simulink model "My_Model"  (R2022a)
settings: Solver=VariableStepAuto  StartTime=0.0  StopTime=10.0  RelTol=1e-3
libraries: neural x1294, spsSeriesRLCBranchLib x16, spsDiodeLib x14, spsMosfetLib x9, spsVoltageMeasurementLib x9, powerlib_extras x8, spsThreePhaseVIMeasurementLib x7, spsCurrentMeasurementLib x4, spsPVArrayLib x4, spsPWMGeneratorDCDCLib x4, spsTHDLib x4, spsThreePhaseParallelRLCBranchLib x3
(part 37 of 41)

== system My_Model/VSC Control/Current Regulator/7 layer network/Layer 4/LW{4,2} ==
  "ad{4,2}" : Inport  PortDimensions=10
      mask Display: e = 0.06;c1 = [120 230 180]/255;c2 = ([120 230 180]+0)/(256+128);c3 = ([120 230 180]+128)/(256+128);patch([0 1 1 0],[0 0 1 1],c1);patch([0 1 1 1-e 1-e 0+e],[0 0 1 1-e 0+e 0+e],c2);patch([0 0 1 1-e 0+e 0+e],[0 1 1 1-e 1-e 0+e],c3);plot([0 1 1 0 0],[0 0 1 1 0]);
  "IW{4,2}(1,:)'" : Constant  Value=[-0.060828921629580597063569058491339092142879962921142578125;0.775373578077013458909050314105115830898284912109375;-1.4812195216760304372627388147520832717418670654296875;1.4414249293693222053747149402624927461147308349609375;-0.600183260490783521134972033905796706676483154296875;-1.0932491360089870990890403845696710050106048583984375;-1.5989219798784224391141606247401796281337738037109375;0.83967493194491271690793610105174593627452850341796875;-1.416112923115345978430923423729836940765380859375;0.90341843686185929751530920839286409318447113037109375]
      mask Display: e = 0.06;c1 = [120 150 230]/255;c2 = ([120 150 230]+0)/383;c3 = ([120 150 230]+128)/383;patch([0 1 1 0],[0 0 1 1],c1);patch([0 1 1 1-e 1-e 0+e],[0 0 1 1-e 0+e 0+e],c2);patch([0 0 1 1-e 0+e 0+e],[0 1 1 1-e 1-e 0+e],c3);plot([0 1 1 0 0],[0 0 1 1 0]);disp('weights');
  "IW{4,2}(10,:)'" : Constant  Value=[0.310879887578999980490834786905907094478607177734375;1.7639693187841471999632858569384552538394927978515625;-0.818751635144346234795875716372393071651458740234375;0.81506969070432278012816595946787856519222259521484375;-1.6295109527652282821463813888840377330780029296875;-0.12293699794713031092641131181153468787670135498046875;-0.72363404737931935617467615884379483759403228759765625;-0.790138494286973358526893207454122602939605712890625;-1.4200799342452998796915153434383682906627655029296875;0.52091465079437615504076575234648771584033966064453125]
      mask Display: e = 0.06;c1 = [120 150 230]/255;c2 = ([120 150 230]+0)/383;c3 = ([120 150 230]+128)/383;patch([0 1 1 0],[0 0 1 1],c1);patch([0 1 1 1-e 1-e 0+e],[0 0 1 1-e 0+e 0+e],c2);patch([0 0 1 1-e 0+e 0+e],[0 1 1 1-e 1-e 0+e],c3);plot([0 1 1 0 0],[0 0 1 1 0]);disp('weights');
  "IW{4,2}(11,:)'" : Constant  Value=[1.217143736034584922123258365900255739688873291015625;0.981955089023607730069898025249131023883819580078125;0.1461353992399598566986895775698940269649028778076171875;0.9371123464038502159922927603474818170070648193359375;-1.095913271537847233361162579967640340328216552734375;1.5274566495244739083858576123020611703395843505859375;-1.586484384110760981201337926904670894145965576171875;0.7160108429212599379098946883459575474262237548828125;0.450020087913313882044263891657465137541294097900390625;0.011825737849426455616796971526127890683710575103759765625]
      mask Display: e = 0.06;c1 = [120 150 230]/255;c2 = ([120 150 230]+0)/383;c3 = ([120 150 230]+128)/383;patch([0 1 1 0],[0 0 1 1],c1);patch([0 1 1 1-e 1-e 0+e],[0 0 1 1-e 0+e 0+e],c2);patch([0 0 1 1-e 0+e 0+e],[0 1 1 1-e 1-e 0+e],c3);plot([0 1 1 0 0],[0 0 1 1 0]);disp('weights');
  "IW{4,2}(12,:)'" : Constant  Value=[1.324541573219643719738769505056552588939666748046875;0.277920776504625433034334491821937263011932373046875;0.718328783591281716525145384366624057292938232421875;-1.42965367074923843659917110926471650600433349609375;0.58329551863306094983130378750502131879329681396484375;-1.3283837730520866582395456134690903127193450927734375;-0.71009288846986395871141439783968962728977203369140625;0.22086308386329200903475111772422678768634796142578125;-0.56919723421407286689799320811289362609386444091796875;-1.1498144669477603496687834194744937121868133544921875]
      mask Display: e = 0.06;c1 = [120 150 230]/255;c2 = ([120 150 230]+0)/383;c3 = ([120 150 230]+128)/383;patch([0 1 1 0],[0 0 1 1],c1);patch([0 1 1 1-e 1-e 0+e],[0 0 1 1-e 0+e 0+e],c2);patch([0 0 1 1-e 0+e 0+e],[0 1 1 1-e 1-e 0+e],c3);plot([0 1 1 0 0],[0 0 1 1 0]);disp('weights');
  "IW{4,2}(13,:)'" : Constant  Value=[1.628084866678424447172801592387259006500244140625;1.46608398126954941886879169032908976078033447265625;-0.03245388683525977924215766279303352348506450653076171875;1.181646003765824293196828875807113945484161376953125;-0.641876045468599887300342743401415646076202392578125;0.82068797136729421115575178191647864878177642822265625;-1.56047384777860198568077976233325898647308349609375;-0.351567530724675225695108338186400942504405975341796875;0.54855116014444627037249802015139721333980560302734375;0.91871473917374724127427043640636838972568511962890625]
      mask Display: e = 0.06;c1 = [120 150 230]/255;c2 = ([120 150 230]+0)/383;c3 = ([120 150 230]+128)/383;patch([0 1 1 0],[0 0 1 1],c1);patch([0 1 1 1-e 1-e 0+e],[0 0 1 1-e 0+e 0+e],c2);patch([0 0 1 1-e 0+e 0+e],[0 1 1 1-e 1-e 0+e],c3);plot([0 1 1 0 0],[0 0 1 1 0]);disp('weights');
  "IW{4,2}(14,:)'" : Constant  Value=[-1.7329463683664869666500862877001054584980010986328125;0.2741436029171386845604274640209041535854339599609375;0.11238014359429461530570648619686835445463657379150390625;1.4837327723600723938801593249081633985042572021484375;1.356169480732644760934135774732567369937896728515625;0.8085467563784864974962829364812932908535003662109375;0.019157902600305108664624498260309337638318538665771484375;-1.519400622506951403778430176316760480403900146484375;0.839192151249030349191571076516993343830108642578125;-1.3888742432581280272785306806326843798160552978515625]
      mask Display: e = 0.06;c1 = [120 150 230]/255;c2 = ([120 150 230]+0)/383;c3 = ([120 150 230]+128)/383;patch([0 1 1 0],[0 0 1 1],c1);patch([0 1 1 1-e 1-e 0+e],[0 0 1 1-e 0+e 0+e],c2);patch([0 0 1 1-e 0+e 0+e],[0 1 1 1-e 1-e 0+e],c3);plot([0 1 1 0 0],[0 0 1 1 0]);disp('weights');
  "IW{4,2}(15,:)'" : Constant  Value=[1.2557485514732544817917414547991938889026641845703125;-1.7036258946208195919069794399547390639781951904296875;-0.1776350386540186676587183001174707897007465362548828125;1.68161376417911156977424980141222476959228515625;-1.33123786422297296638816987979225814342498779296875;0.22183289060876243414810460308217443525791168212890625;0.92045836890086685233569596675806678831577301025390625;0.9665236347790635562660099822096526622772216796875;0.31881726521650388672668441358837299048900604248046875;-0.7597052386250791045085861696861684322357177734375]
      mask Display: e = 0.06;c1 = [120 150 230]/255;c2 = ([120 150 230]+0)/383;c3 = ([120 150 230]+128)/383;patch([0 1 1 0],[0 0 1 1],c1);patch([0 1 1 1-e 1-e 0+e],[0 0 1 1-e 0+e 0+e],c2);patch([0 0 1 1-e 0+e 0+e],[0 1 1 1-e 1-e 0+e],c3);plot([0 1 1 0 0],[0 0 1 1 0]);disp('weights');
  "IW{4,2}(16,:)'" : Constant  Value=[0.383590307363950333563451522422838024795055389404296875;-1.441254533680973448639406342408619821071624755859375;-1.404217028320909665950466660433448851108551025390625;1.378999030353992960584719185135327279567718505859375;1.8023155948177276286514825187623500823974609375;-1.17934167700769165776364388875663280487060546875;0.46513754528094886087075110481237061321735382080078125;-0.61955378906156199914079252266674302518367767333984375;0.87675658573421488828358860700973309576511383056640625;-1.0257452924889649548134684664546512067317962646484375]
      mask Display: e = 0.06;c1 = [120 150 230]/255;c2 = ([120 150 230]+0)/383;c3 = ([120 150 230]+128)/383;patch([0 1 1 0],[0 0 1 1],c1);patch([0 1 1 1-e 1-e 0+e],[0 0 1 1-e 0+e 0+e],c2);patch([0 0 1 1-e 0+e 0+e],[0 1 1 1-e 1-e 0+e],c3);plot([0 1 1 0 0],[0 0 1 1 0]);disp('weights');
  "IW{4,2}(17,:)'" : Constant  Value=[2.16839681738434553182059971732087433338165283203125;1.6098123671258501854453015766921453177928924560546875;-0.0775879150485726809538533643717528320848941802978515625;1.246473799287855843687111701001413166522979736328125;0.131071502196153488739582826383411884307861328125;0.437504287344965214767711358945234678685665130615234375;-1.819738309523170727288743364624679088592529296875;0.4628385267851713447129213818698190152645111083984375;-1.22740730807900977339386372477747499942779541015625;0.118226785158787262020041453070007264614105224609375]
      mask Display: e = 0.06;c1 = [120 150 230]/255;c2 = ([120 150 230]+0)/383;c3 = ([120 150 230]+128)/383;patch([0 1 1 0],[0 0 1 1],c1);patch([0 1 1 1-e 1-e 0+e],[0 0 1 1-e 0+e 0+e],c2);patch([0 0 1 1-e 0+e 0+e],[0 1 1 1-e 1-e 0+e],c3);plot([0 1 1 0 0],[0 0 1 1 0]);disp('weights');
  "IW{4,2}(18,:)'" : Constant  Value=[0.107059477512987777370057074222131632268428802490234375;-0.06585053325048302597100047250933130271732807159423828125;1.4630069984471634203515577610232867300510406494140625;0.0477064948285615686440763738573878072202205657958984375;0.85086691079940413029447654480463825166225433349609375;-0.828227053520045775059088555281050503253936767578125;-1.73790831566754011561215520487166941165924072265625;0.990421071262879149088576014037244021892547607421875;0.97314868113544061856146072386763989925384521484375;-1.7005202976191835517738581984303891658782958984375]
      mask Display: e = 0.06;c1 = [120 150 230]/255;c2 = ([120 150 230]+0)/383;c3 = ([120 150 230]+128)/383;patch([0 1 1 0],[0 0 1 1],c1);patch([0 1 1 1-e 1-e 0+e],[0 0 1 1-e 0+e 0+e],c2);patch([0 0 1 1-e 0+e 0+e],[0 1 1 1-e 1-e 0+e],c3);plot([0 1 1 0 0],[0 0 1 1 0]);disp('weights');
  "IW{4,2}(19,:)'" : Constant  Value=[-0.1068335199342358154961374339109170250594615936279296875;1.213999003127531839396624491200782358646392822265625;1.280461050341758610926490291603840887546539306640625;-1.1633486924833695841385861058370210230350494384765625;1.714241791837474604420776813640259206295013427734375;-1.2950432592145111332371243406669236719608306884765625;0.98042672986934353840382527778274379670619964599609375;-1.4085702082696258674587852510740049183368682861328125;1.6061426617917649029010362937697209417819976806640625;-0.369230851288646355623512818056042306125164031982421875]
      mask Display: e = 0.06;c1 = [120 150 230]/255;c2 = ([120 150 230]+0)/383;c3 = ([120 150 230]+128)/383;patch([0 1 1 0],[0 0 1 1],c1);patch([0 1 1 1-e 1-e 0+e],[0 0 1 1-e 0+e 0+e],c2);patch([0 0 1 1-e 0+e 0+e],[0 1 1 1-e 1-e 0+e],c3);plot([0 1 1 0 0],[0 0 1 1 0]);disp('weights');
  "IW{4,2}(2,:)'" : Constant  Value=[-1.0650580520005401563565783362719230353832244873046875;0.290106267548429330727088881758390925824642181396484375;-0.0626025735426334606348319766766508109867572784423828125;-1.4192383868717663997216504867537878453731536865234375;-0.1107366893851524647374162668711505830287933349609375;-0.479209457315004250244072636633063666522502899169921875;1.3599037924116783582206835490069352090358734130859375;-1.695981597854835598582212696783244609832763671875;-1.5234679846656782320479806003277190029621124267578125;-0.456163743131432208866016253523412160575389862060546875]
      mask Display: e = 0.06;c1 = [120 150 230]/255;c2 = ([120 150 230]+0)/383;c3 = ([120 150 230]+128)/383;patch([0 1 1 0],[0 0 1 1],c1);patch([0 1 1 1-e 1-e 0+e],[0 0 1 1-e 0+e 0+e],c2);patch([0 0 1 1-e 0+e 0+e],[0 1 1 1-e 1-e 0+e],c3);plot([0 1 1 0 0],[0 0 1 1 0]);disp('weights');
  "IW{4,2}(20,:)'" : Constant  Value=[1.0166778965638318954489704992738552391529083251953125;-0.98714156775735439897090373051469214260578155517578125;-0.7796210586513101503669531666673719882965087890625;-0.343692816023216718424038162993383593857288360595703125;-0.72737705933559271276322988342144526541233062744140625;-0.974145375754890796571316968766041100025177001953125;1.3709769292688307462668717562337405979633331298828125;-1.263090823913412652501619959366507828235626220703125;1.24527862717969117767324860324151813983917236328125;-1.346273420594027658836466798675246536731719970703125]
      mask Display: e = 0.06;c1 = [120 150 230]/255;c2 = ([120 150 230]+0)/383;c3 = ([120 150 230]+128)/383;patch([0 1 1 0],[0 0 1 1],c1);patch([0 1 1 1-e 1-e 0+e],[0 0 1 1-e 0+e 0+e],c2);patch([0 0 1 1-e 0+e 0+e],[0 1 1 1-e 1-e 0+e],c3);plot([0 1 1 0 0],[0 0 1 1 0]);disp('weights');
  "IW{4,2}(21,:)'" : Constant  Value=[-1.1458486736864827992832260861177928745746612548828125;0.2200149413124674879771447422172059305012226104736328125;-1.22701113163355568502765891025774180889129638671875;-1.5407070305327781323256886025774292647838592529296875;-0.36019231507982940598822096944786608219146728515625;1.6621539392872619611551954221795313060283660888671875;0.1419004661333211902984885455225594341754913330078125;0.2082746842913306972722153886934393085539340972900390625;-1.741546190079789280247268834500573575496673583984375;-1.632095283173258248865522546111606061458587646484375]
      mask Display: e = 0.06;c1 = [120 150 230]/255;c2 = ([120 150 230]+0)/383;c3 = ([120 150 230]+128)/383;patch([0 1 1 0],[0 0 1 1],c1);patch([0 1 1 1-e 1-e 0+e],[0 0 1 1-e 0+e 0+e],c2);patch([0 0 1 1-e 0+e 0+e],[0 1 1 1-e 1-e 0+e],c3);plot([0 1 1 0 0],[0 0 1 1 0]);disp('weights');
  "IW{4,2}(22,:)'" : Constant  Value=[0.051518019703444994927821198871242813766002655029296875;0.449024556110029171573927442295826040208339691162109375;0.278527593749954949231550926924683153629302978515625;-1.5469829135579071799355688199284486472606658935546875;-0.06756097927501138189487761565032997168600559234619140625;-1.4415773126596402864407764354837127029895782470703125;-1.341684335449111475924155456596054136753082275390625;-0.027032608761643601991142560336811584420502185821533203125;-0.453046390752525007794559996909811161458492279052734375;1.0339124076123431539286912084207870066165924072265625]
      mask Display: e = 0.06;c1 = [120 150 230]/255;c2 = ([120 150 230]+0)/383;c3 = ([120 150 230]+128)/383;patch([0 1 1 0],[0 0 1 1],c1);patch([0 1 1 1-e 1-e 0+e],[0 0 1 1-e 0+e 0+e],c2);patch([0 0 1 1-e 0+e 0+e],[0 1 1 1-e 1-e 0+e],c3);plot([0 1 1 0 0],[0 0 1 1 0]);disp('weights');
  "IW{4,2}(23,:)'" : Constant  Value=[1.410523325508492131774573863367550075054168701171875;-1.6502033117988690325006473358371295034885406494140625;0.49454814607619013155925813407520763576030731201171875;1.547650452106767549054211485781706869602203369140625;0.930327812469440740272830225876532495021820068359375;-0.9081222480249990791634218112449161708354949951171875;1.1479814503964977934202806864050216972827911376953125;1.3759059769361836611523131068679504096508026123046875;-0.461553991984265998826941768129472620785236358642578125;-0.737241361510495352149519021622836589813232421875]
      mask Display: e = 0.06;c1 = [120 150 230]/255;c2 = ([120 150 230]+0)/383;c3 = ([120 150 230]+128)/383;patch([0 1 1 0],[0 0 1 1],c1);patch([0 1 1 1-e 1-e 0+e],[0 0 1 1-e 0+e 0+e],c2);patch([0 0 1 1-e 0+e 0+e],[0 1 1 1-e 1-e 0+e],c3);plot([0 1 1 0 0],[0 0 1 1 0]);disp('weights');
  "IW{4,2}(24,:)'" : Constant  Value=[0.28120223249780063046188161024474538862705230712890625;0.431184756844114669416256901968154124915599822998046875;-0.3114845912627794977112216656678356230258941650390625;-0.74778874942729967045806915848515927791595458984375;1.1960256549365488876190966038848273456096649169921875;-1.67696123599303792417458680574782192707061767578125;-0.6073695589822538654090067211654968559741973876953125;1.123864797023088168970161859760992228984832763671875;0.69580073511743723013722728865104727447032928466796875;0.3893164178598220726001954972161911427974700927734375]
      mask Display: e = 0.06;c1 = [120 150 230]/255;c2 = ([120 150 230]+0)/383;c3 = ([120 150 230]+128)/383;patch([0 1 1 0],[0 0 1 1],c1);patch([0 1 1 1-e 1-e 0+e],[0 0 1 1-e 0+e 0+e],c2);patch([0 0 1 1-e 0+e 0+e],[0 1 1 1-e 1-e 0+e],c3);plot([0 1 1 0 0],[0 0 1 1 0]);disp('weights');
  "IW{4,2}(25,:)'" : Constant  Value=[1.1045182165218836445319539052434265613555908203125;-0.4482836953092930176723029944696463644504547119140625;-0.95651367760070693524454554790281690657138824462890625;-0.66727478432028386468033431810908950865268707275390625;-1.30390522059007007982245340826921164989471435546875;-0.1900347355466538157298117539539816789329051971435546875;-0.6732421716764174224323369344347156584262847900390625;0.75538737318340187787413242403999902307987213134765625;0.306495894053974649029470356254023499786853790283203125;1.4935364929146019985495286164223216474056243896484375]
      mask Display: e = 0.06;c1 = [120 150 230]/255;c2 = ([120 150 230]+0)/383;c3 = ([120 150 230]+128)/383;patch([0 1 1 0],[0 0 1 1],c1);patch([0 1 1 1-e 1-e 0+e],[0 0 1 1-e 0+e 0+e],c2);patch([0 0 1 1-e 0+e 0+e],[0 1 1 1-e 1-e 0+e],c3);plot([0 1 1 0 0],[0 0 1 1 0]);disp('weights');
  "IW{4,2}(3,:)'" : Constant  Value=[0.00050827964445552338730582864201323900488205254077911376953125;-0.81647006445067804580872916631051339209079742431640625;-0.975377897978984886862008352181874215602874755859375;-1.25948524250642268640376641997136175632476806640625;0.495526011700579027685620303600444458425045013427734375;-1.4322750685215390742399677037610672414302825927734375;-0.98115044653176253230952852391055785119533538818359375;-1.4443199539421411881079393424442969262599945068359375;-1.3135393988054457903302818522206507623195648193359375;-0.93411089648263512241754824572126381099224090576171875]
      mask Display: e = 0.06;c1 = [120 150 230]/255;c2 = ([120 150 230]+0)/383;c3 = ([120 150 230]+128)/383;patch([0 1 1 0],[0 0 1 1],c1);patch([0 1 1 1-e 1-e 0+e],[0 0 1 1-e 0+e 0+e],c2);patch([0 0 1 1-e 0+e 0+e],[0 1 1 1-e 1-e 0+e],c3);plot([0 1 1 0 0],[0 0 1 1 0]);disp('weights');
  "IW{4,2}(4,:)'" : Constant  Value=[-1.193085532573731288863427835167385637760162353515625;0.58746447103715671023138611417380161583423614501953125;-1.297431094068265178265164649928919970989227294921875;-1.2225716771040604502474025139235891401767730712890625;-1.6233857883220110807087621651589870452880859375;0.046795075748082483324541414049235754646360874176025390625;-1.395408461889833251490244947490282356739044189453125;0.634455127417530295730330180958844721317291259765625;1.0230197707863570855124635272659361362457275390625;-1.4104901214324545577483149827457964420318603515625]
      mask Display: e = 0.06;c1 = [120 150 230]/255;c2 = ([120 150 230]+0)/383;c3 = ([120 150 230]+128)/383;patch([0 1 1 0],[0 0 1 1],c1);patch([0 1 1 1-e 1-e 0+e],[0 0 1 1-e 0+e 0+e],c2);patch([0 0 1 1-e 0+e 0+e],[0 1 1 1-e 1-e 0+e],c3);plot([0 1 1 0 0],[0 0 1 1 0]);disp('weights');
  "IW{4,2}(5,:)'" : Constant  Value=[-1.5064865353503862355211140311439521610736846923828125;-1.4094825613739774272659133202978409826755523681640625;-0.99730592434702047821559744988917373120784759521484375;-1.1293501614278047551209738230681978166103363037109375;1.157186358015720006875426406622864305973052978515625;-0.555516378672133104288377580814994871616363525390625;-0.65180464082589484320351402857340872287750244140625;0.349564186768515805514567773570888675749301910400390625;1.4984956166963794288449207670055329799652099609375;0.91950057800333440116702377054025419056415557861328125]
      mask Display: e = 0.06;c1 = [120 150 230]/255;c2 = ([120 150 230]+0)/383;c3 = ([120 150 230]+128)/383;patch([0 1 1 0],[0 0 1 1],c1);patch([0 1 1 1-e 1-e 0+e],[0 0 1 1-e 0+e 0+e],c2);patch([0 0 1 1-e 0+e 0+e],[0 1 1 1-e 1-e 0+e],c3);plot([0 1 1 0 0],[0 0 1 1 0]);disp('weights');
  "IW{4,2}(6,:)'" : Constant  Value=[1.2867800822025874385445831649121828377246856689453125;0.461592629060466830281939110136590898036956787109375;-1.2934705271869806342266429055598564445972442626953125;0.444150757716133048891293810811475850641727447509765625;0.218196104926050737926601641447632573544979095458984375;-1.1872371945991611053017322774394415318965911865234375;-0.161186428964905648086869405233301222324371337890625;0.09811372829240284920704340265729115344583988189697265625;0.67645667782540652712697237802785821259021759033203125;-1.07525627614175522950290542212314903736114501953125]
      mask Display: e = 0.06;c1 = [120 150 230]/255;c2 = ([120 150 230]+0)/383;c3 = ([120 150 230]+128)/383;patch([0 1 1 0],[0 0 1 1],c1);patch([0 1 1 1-e 1-e 0+e],[0 0 1 1-e 0+e 0+e],c2);patch([0 0 1 1-e 0+e 0+e],[0 1 1 1-e 1-e 0+e],c3);plot([0 1 1 0 0],[0 0 1 1 0]);disp('weights');
  "IW{4,2}(7,:)'" : Constant  Value=[0.2754985337353932361992292499053291976451873779296875;0.5930221081919075931665474854526109993457794189453125;-1.0930149653653142838294343164307065308094024658203125;0.32612797438859997267712742541334591805934906005859375;1.360263389427888380822651015478186309337615966796875;-1.0580489451859786953491493477486073970794677734375;-1.4699115220963008265897542514721862971782684326171875;0.89389866993477273826584905691561289131641387939453125;-1.3208420362101145340005814432515762746334075927734375;-0.3598583784269588914384030431392602622509002685546875]
      mask Display: e = 0.06;c1 = [120 150 230]/255;c2 = ([120 150 230]+0)/383;c3 = ([120 150 230]+128)/383;patch([0 1 1 0],[0 0 1 1],c1);patch([0 1 1 1-e 1-e 0+e],[0 0 1 1-e 0+e 0+e],c2);patch([0 0 1 1-e 0+e 0+e],[0 1 1 1-e 1-e 0+e],c3);plot([0 1 1 0 0],[0 0 1 1 0]);disp('weights');
  "IW{4,2}(8,:)'" : Constant  Value=[1.252291948767795926045209853327833116054534912109375;0.684639083059272568476671949611045420169830322265625;-1.3886367035327016328238869391498155891895294189453125;-1.377726677378242836624622214003466069698333740234375;-0.49335075352307422580366846887045539915561676025390625;1.1994100753566210304512651418917812407016754150390625;1.4910277439208845517981671946472488343715667724609375;0.611513604974813329562266517314128577709197998046875;0.65411948575318523690924621405429206788539886474609375;0.11907554098075810722345835301894112490117549896240234375]
      mask Display: e = 0.06;c1 = [120 150 230]/255;c2 = ([120 150 230]+0)/383;c3 = ([120 150 230]+128)/383;patch([0 1 1 0],[0 0 1 1],c1);patch([0 1 1 1-e 1-e 0+e],[0 0 1 1-e 0+e 0+e],c2);patch([0 0 1 1-e 0+e 0+e],[0 1 1 1-e 1-e 0+e],c3);plot([0 1 1 0 0],[0 0 1 1 0]);disp('weights');
  "IW{4,2}(9,:)'" : Constant  Value=[0.72630368095153585716872157718171365559101104736328125;1.513729352522219517851453929324634373188018798828125;0.50942637936254164809923850043560378253459930419921875;1.640606006877881828387444329564459621906280517578125;-0.251485920263373519123462074276176281273365020751953125;0.6621978703362703111423570589977316558361053466796875;-0.64239933964905693297708921818411909043788909912109375;1.1005966289439366168068090701126493513584136962890625;-1.521958129733803399830094349454157054424285888671875;-1.09241515202251004978961645974777638912200927734375]
      mask Display: e = 0.06;c1 = [120 150 230]/255;c2 = ([120 150 230]+0)/383;c3 = ([120 150 230]+128)/383;patch([0 1 1 0],[0 0 1 1],c1);patch([0 1 1 1-e 1-e 0+e],[0 0 1 1-e 0+e 0+e],c2);patch([0 0 1 1-e 0+e 0+e],[0 1 1 1-e 1-e 0+e],c3);plot([0 1 1 0 0],[0 0 1 1 0]);disp('weights');
  Mux : Mux  Inputs=25
      mask Display: e = 0.06;c1 = [120 150 230]/255;c2 = ([120 150 230]+0)/383;c3 = ([120 150 230]+128)/383;patch([0 1 1 0],[0 0 1 1],c1);patch([0 1 1 1-e 1-e 0+e],[0 0 1 1-e 0+e 0+e],c2);patch([0 0 1 1-e 0+e 0+e],[0 1 1 1-e 1-e 0+e],c3);plot([0 1 1 0 0],[0 0 1 1 0]);disp('Mux');
  dotprod{1..25} (25 alike) : neural/Weight Functions/dotprod
  "lz{4,2}" : Outport
      mask Display: e = 0.06;c1 = [120 230 180]/255;c2 = ([120 230 180]+0)/(256+128);c3 = ([120 230 180]+128)/(256+128);patch([0 1 1 0],[0 0 1 1],c1);patch([0 1 1 1-e 1-e 0+e],[0 0 1 1-e 0+e 0+e],c2);patch([0 0 1 1-e 0+e 0+e],[0 1 1 1-e 1-e 0+e],c3);plot([0 1 1 0 0],[0 0 1 1 0]);
  wires:
  "IW{4,2}(1,:)'"/1 -> dotprod1/1
  "ad{4,2}"/1 -> dotprod1/2, dotprod2/2, dotprod3/2, dotprod4/2, dotprod5/2, dotprod6/2, dotprod7/2, dotprod8/2, dotprod9/2, dotprod10/2, dotprod11/2, dotprod12/2, dotprod13/2, dotprod14/2, dotprod15/2, dotprod16/2, dotprod17/2, dotprod18/2, dotprod19/2, dotprod20/2, dotprod21/2, dotprod22/2, dotprod23/2, dotprod24/2, dotprod25/2
  dotprod1/1 -> Mux/1
  "IW{4,2}(2,:)'"/1 -> dotprod2/1
  dotprod2/1 -> Mux/2
  "IW{4,2}(3,:)'"/1 -> dotprod3/1
  dotprod3/1 -> Mux/3
  "IW{4,2}(4,:)'"/1 -> dotprod4/1
  dotprod4/1 -> Mux/4
  "IW{4,2}(5,:)'"/1 -> dotprod5/1
  dotprod5/1 -> Mux/5
  "IW{4,2}(6,:)'"/1 -> dotprod6/1
  dotprod6/1 -> Mux/6
  "IW{4,2}(7,:)'"/1 -> dotprod7/1
  dotprod7/1 -> Mux/7
  "IW{4,2}(8,:)'"/1 -> dotprod8/1
  dotprod8/1 -> Mux/8
  "IW{4,2}(9,:)'"/1 -> dotprod9/1
  dotprod9/1 -> Mux/9
  "IW{4,2}(10,:)'"/1 -> dotprod10/1
  dotprod10/1 -> Mux/10
  "IW{4,2}(11,:)'"/1 -> dotprod11/1
  dotprod11/1 -> Mux/11
  "IW{4,2}(12,:)'"/1 -> dotprod12/1
  dotprod12/1 -> Mux/12
  "IW{4,2}(13,:)'"/1 -> dotprod13/1
  dotprod13/1 -> Mux/13
  "IW{4,2}(14,:)'"/1 -> dotprod14/1
  dotprod14/1 -> Mux/14
  "IW{4,2}(15,:)'"/1 -> dotprod15/1
  dotprod15/1 -> Mux/15
  "IW{4,2}(16,:)'"/1 -> dotprod16/1
  dotprod16/1 -> Mux/16
  "IW{4,2}(17,:)'"/1 -> dotprod17/1
  dotprod17/1 -> Mux/17
  "IW{4,2}(18,:)'"/1 -> dotprod18/1
  dotprod18/1 -> Mux/18
  "IW{4,2}(19,:)'"/1 -> dotprod19/1
  dotprod19/1 -> Mux/19
  "IW{4,2}(20,:)'"/1 -> dotprod20/1
  dotprod20/1 -> Mux/20
  "IW{4,2}(21,:)'"/1 -> dotprod21/1
  dotprod21/1 -> Mux/21
  "IW{4,2}(22,:)'"/1 -> dotprod22/1
  dotprod22/1 -> Mux/22
  "IW{4,2}(23,:)'"/1 -> dotprod23/1
  dotprod23/1 -> Mux/23
  "IW{4,2}(24,:)'"/1 -> dotprod24/1
  dotprod24/1 -> Mux/24
  "IW{4,2}(25,:)'"/1 -> dotprod25/1
  dotprod25/1 -> Mux/25
  Mux/1 -> "lz{4,2}"/1
